simulink model "hw1_acc_model2"  (R2017a)
settings: Solver=ode45  StartTime=0.0  StopTime=15  RelTol=1e-3  EnableMultiTasking=on
InitFcn:
  | m = 1000;
  | b = 50;
libraries: simulink x1
settings Model: Creator=edward  LastModifiedBy=edward
settings DataIOCC: LimitDataPoints=on  SaveFormat=Array
settings OptimizationCC: LifeSpan=inf
settings DebuggingCC: UnderspecifiedInitializationDetection=Classic  MergeDetectMultiDrivingBlocksExec=none  SolverPrmCheckMsg=warning  SFUnexpectedBacktrackingDiag=warning  SFNoUnconditionalDefaultTransitionDiag=warning  SFExecutionAtInitializationDiag=none
settings HardwareCC: ProdBitPerPointer=32  ProdBitPerSizeT=32  ProdBitPerPtrDiffT=32  ProdLargestAtomicFloat=None  ProdIntDivRoundTo=Undefined  ProdEndianess=Unspecified  ProdWordSize=32  ProdHWDeviceType=32-bit Generic
settings ModelReferenceCC: PropagateSignalLabelsOutOfModel=off
settings GRTTargetCC: TargetLangStandard=C89/C90 (ANSI)  GeneratePreprocessorConditionals=Disable all
settings ConfigComp: CovMetricSettings=dw  CovHtmlReporting=on  CovSaveCumulativeToWorkspaceVar=on  CovSaveSingleToWorkspaceVar=on  CovExternalEMLEnable=off

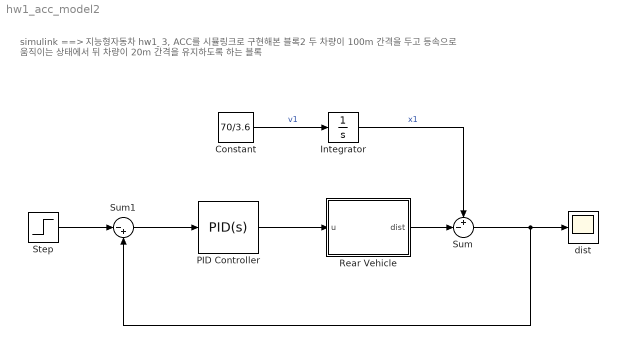
== system hw1_acc_model2 ==
  note: simulink ==> 지능형자동차 hw1_3, ACC를 시뮬링크로 구현해본 블록2
      | 두 차량이 100m 간격을 두고 등속으로 움직이는 상태에서
      | 뒤 차량이 20m 간격을 유지하도록 하는 블록
  Constant : Constant  Value=70/3.6
  Integrator : Integrator  InitialCondition=100
  PID Controller : simulink/Continuous/PID Controller  Controller=PID  TimeDomain=Continuous-time  SampleTime=-1  IntegratorMethod=Forward Euler  FilterMethod=Forward Euler  Form=Parallel  UseFilter=on  ControllerParametersSource=internal  P=1000  I=10  D=1500  N=100  InitialConditionSource=internal  InitialConditionForIntegrator=0  InitialConditionForFilter=0  ExternalReset=none  LimitOutput=off  UpperSaturationLimit=inf  LowerSaturationLimit=-inf  LinearizeAsGain=on  AntiWindupMode=none  Kb=1  TrackingMode=off  Kt=1  PParamMin=[]  PParamMax=[]  IParamMin=[]  IParamMax=[]  DParamMin=[]  DParamMax=[]  NParamMin=[]  NParamMax=[]  KbParamMin=[]  KbParamMax=[]  KtParamMin=[]  KtParamMax=[]  POutMin=[]  POutMax=[]  IOutMin=[]  IOutMax=[]  DOutMin=[]  DOutMax=[]  NOutMin=[]  NOutMax=[]  KbOutMin=[]  KbOutMax=[]  KtOutMin=[]  KtOutMax=[]  IntegratorOutMin=[]  IntegratorOutMax=[]  FilterOutMin=[]  FilterOutMax=[]  SumOutMin=[]  SumOutMax=[]  SumI1OutMin=[]  SumI1OutMax=[]  SumI2OutMin=[]  SumI2OutMax=[]  SumI3OutMin=[]  SumI3OutMax=[]  SumDOutMin=[]  SumDOutMax=[]  SaturationOutMin=[]  SaturationOutMax=[]  IntegratorContinuousStateAttributes=''  IntegratorStateMustResolveToSignalObject=off  IntegratorRTWStateStorageClass=Auto  FilterContinuousStateAttributes=''  FilterStateMustResolveToSignalObject=off  FilterRTWStateStorageClass=Auto  DifferentiatorICPrevScaledInput=0  DifferentiatorOutMin=[]  DifferentiatorOutMax=[]  InitialConditionSetting=State (most efficient)
  Rear Vehicle : Subsystem
  Step : Step  Time=0  After=20  SampleTime=0
  Sum : Sum  Inputs=+-|
  Sum1 : Sum  Inputs=|-+
  dist : Scope
  wires:
  PID Controller/1 -> Rear Vehicle/1(u)
  Constant/1 -> Integrator/1  "v1"
  Integrator/1 -> Sum/1  "x1"
  Rear Vehicle/1(dist) -> Sum/2
  Sum/1 -> Sum1/2, dist/1
  Sum1/1 -> PID Controller/1
  Step/1 -> Sum1/1

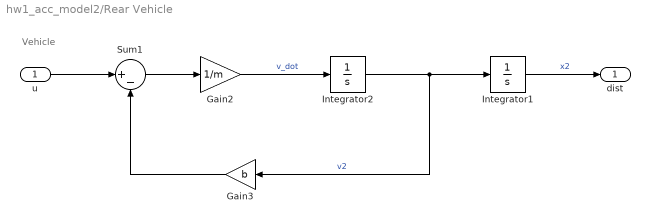
== system hw1_acc_model2/Rear Vehicle ==
  note: Vehicle
  u : Inport
  Gain2 : Gain  Gain=1/m
  Gain3 : Gain  Gain=b
  Integrator1 : Integrator
  Integrator2 : Integrator  InitialCondition=70/3.6
  Sum1 : Sum  Inputs=|+-
  dist : Outport
  wires:
  u/1 -> Sum1/1
  Integrator2/1 -> Integrator1/1, Gain3/1  "v2"
  Sum1/1 -> Gain2/1
  Gain2/1 -> Integrator2/1  "v_dot"
  Gain3/1 -> Sum1/2
  Integrator1/1 -> dist/1  "x2"
